simulink model "DC_SpeedControl"  (R2019b)
settings: Solver=VariableStepAuto  StartTime=0.0  StopTime=inf  RelTol=1e-3
libraries: powerlib x11, simulink x1
settings Model: Creator=Admin  LastModifiedBy=DELL
settings DataIOCC: ReturnWorkspaceOutputs=off
settings DebuggingCC: ArithmeticOperatorsInVariantConditions=warning
settings SFSimCC: SimUseLocalCustomCode=off  CustomCodeUndefinedFunction=UseInterfaceOnly
settings RTWCC: RTWUseLocalCustomCode=off

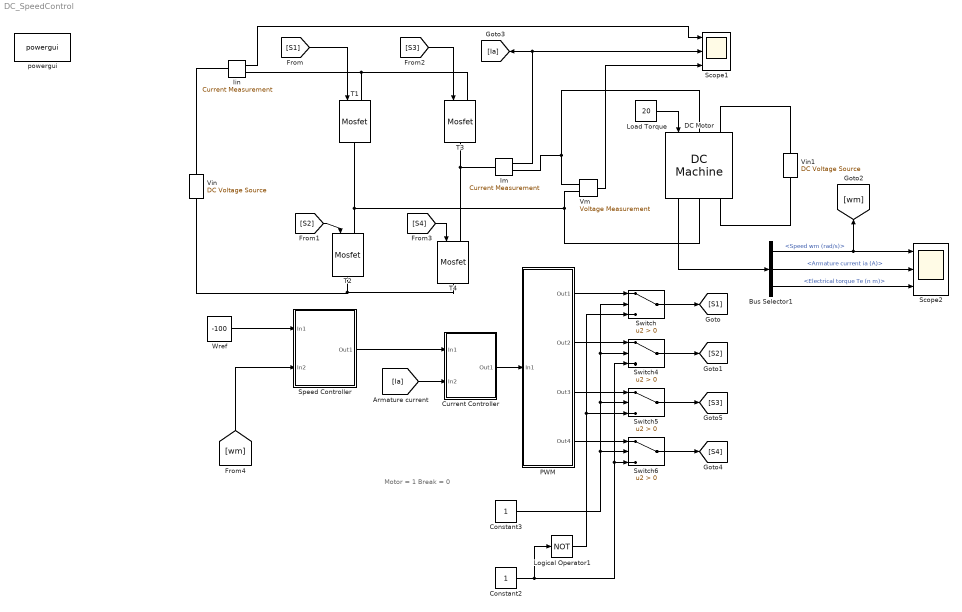
== system DC_SpeedControl ==
  note: Motor = 1
      | Break = 0
  Bus Selector1 : BusSelector  OutputSignals=Speed wm (rad/s),Armature current ia (A),Electrical torque Te (n m)
  Constant2 : Constant
  Constant3 : Constant
  Current Controller : Subsystem
  DC Motor : powerlib/Machines/DC Machine  PresetModel=02: 5HP 240V 1750RPM Field:150V  MechanicalLoad=Torque TL  FieldType=Wound  ShowDetailedParameters=on  MeasurementBus=off  RLa=[0.78 0.016]  RLf=[150 112.5]  Laf=1.234  MachineConstant=Torque constant (N.m/A)  Ke=1.8  Kt=1.8  J=0.05  Bm=0.01  Tf=0  w0=1  Ifinit=1  TsPowergui=0  TsBlock=-1
      settings: SourceProductName=Simscape Electrical
  Iin : powerlib/Measurements/Current Measurement  PhasorSimulation=off  OutputType=Complex  PSBequivalent=0
      settings: SourceProductName=Simscape Electrical
  Im : powerlib/Measurements/Current Measurement  PhasorSimulation=off  OutputType=Complex  PSBequivalent=0
      settings: SourceProductName=Simscape Electrical
  Load Torque : Constant  Value=20
  Logical Operator1 : Logic  Operator=NOT  AllPortsSameDT=off  OutDataTypeStr=boolean
  PWM : Subsystem
  Scope1 : Scope  NumInputPorts=3
  Scope2 : Scope  NumInputPorts=3
  Speed Controller : Subsystem
  Switch{,4..6} (4 alike) : Switch  Criteria=u2 > Threshold
  T{1..4} (4 alike) : powerlib/Power Electronics/Mosfet  Ron=0.1  Lon=0  Rd=0.01  Vfd=0  IC=0  Rs=1e5  Cs=inf  Measurements=off
      settings: SourceProductName=Simscape Electrical
  Vin : powerlib/Electrical Sources/DC Voltage Source  Amplitude=300  Measurements=None
      settings: SourceProductName=Simscape Electrical
  Vin1 : powerlib/Electrical Sources/DC Voltage Source  Amplitude=150  Measurements=None
      settings: SourceProductName=Simscape Electrical
  Vm : powerlib/Measurements/Voltage Measurement  PhasorSimulation=off  OutputType=Complex  PSBequivalent=0
      settings: SourceProductName=Simscape Electrical
  Wref : Constant  Value=-100  VectorParams1D=off  SampleTime=-1
  powergui : powerlib/powergui  Priority=1  SimulationMode=Continuous  SampleTime=50e-6  frequency=60  Iterations=50  frequencyindice=0  Pbase=100e6  ErrMax=1e-4  UnitsV=kV  UnitsW=MW  buscounter=0  FunctionMessages=off  echomessages=off  EnableUseOfTLC=off  CurrentSourceSwitches=off  DisableSnubberDevices=off  DisableRonSwitches=off  DisableVfSwitches=off  DisplayEquations=off  AutomaticDiscreteSolvers=off  SolverType=Tustin/Backward Euler (TBE)  Interpol=off  ExternalGateDelay=off  methode=off  Ts=100  x0status=blocks  SPID=on  SwTol=0  HookPort=off  NonlinearTolerance=1e-4  nMaxIteration=100  ContinueOnMaxIteration=off  RestoreLinks=warning  ResistiveCurrentMeasurement=off  Frange=[0:2:500]  Ylog=off  Xlog=on  ShowGrid=off  save=off  variable=ZData  structure=0  ZoomFFT=off  StartTime=0.0  cycles=1  DisplayStyle=1  fundamental=60  FreqAxis=off  MaxFrequency=1000  frequencyindicesteady=1  RmsSteady=1  display=off
      settings: SourceProductName=Simscape Electrical
  wires:
  Vm/1 -> Scope1/3
  Bus Selector1/1 -> [wm], Scope2/1  "<Speed wm (rad/s)>"
  Load Torque/1 -> DC Motor/1
  Bus Selector1/2 -> Scope2/2  "<Armature current ia (A)>"
  Iin/1 -> Scope1/1
  [S1] -> T1/1
  Bus Selector1/3 -> Scope2/3  "<Electrical torque Te (n m)>"
  [S3] -> T3/1
  DC Motor/1 -> Bus Selector1/1
  Im/1 -> [Ia], Scope1/2
  Wref/1 -> Speed Controller/1(In1)
  Speed Controller/1(Out1) -> Current Controller/1(In1)
  [Ia] -> Current Controller/2(In2)
  Current Controller/1(Out1) -> PWM/1(In1)
  [S4] -> T4/1
  [S2] -> T2/1
  PWM/1(Out1) -> Switch/1
  Switch/1 -> [S1]
  PWM/2(Out2) -> Switch4/1
  Switch4/1 -> [S2]
  PWM/3(Out3) -> Switch5/1
  Switch5/1 -> [S3]
  PWM/4(Out4) -> Switch6/1
  Switch6/1 -> [S4]
  Constant3/1 -> Switch5/2, Switch4/2, Switch/2, Switch6/2
  Constant2/1 -> Switch6/3, Switch4/3, Logical Operator1/1
  Logical Operator1/1 -> Switch5/3, Switch/3
  [wm] -> Speed Controller/2(In2)
  connections:
  T1/RConn1 -- Vm/LConn2 -- DC Motor/RConn1 -- T2/LConn1
  Im/RConn1 -- Vm/LConn1 -- DC Motor/LConn1
  Iin/RConn1 -- T1/LConn1 -- T3/LConn1
  Vin/LConn1 -- T4/RConn1 -- T2/RConn1
  Vin1/LConn1 -- DC Motor/RConn2
  Iin/LConn1 -- Vin/RConn1
  DC Motor/LConn2 -- Vin1/RConn1
  T4/LConn1 -- T3/RConn1 -- Im/LConn1

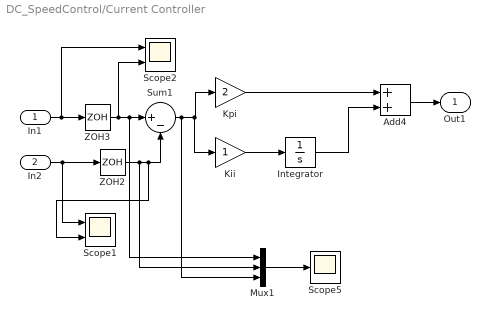
== system DC_SpeedControl/Current Controller ==
  In1 : Inport
  In2 : Inport  Port=2
  Add4 : Sum
  Integrator : Integrator
  Kii : Gain
  Kpi : Gain  Gain=2
  Mux1 : Mux  Inputs=3
  Scope1 : Scope  NumInputPorts=2
  Scope2 : Scope  NumInputPorts=2
  Scope5 : Scope
  Sum1 : Sum  Inputs=|+-
  ZOH2 : ZeroOrderHold  SampleTime=1e-4
  ZOH3 : ZeroOrderHold  SampleTime=1e-4
  Out1 : Outport  VectorParamsAs1DForOutWhenUnconnected=off
  wires:
  ZOH3/1 -> Scope2/2, Mux1/1, Sum1/1
  Kii/1 -> Integrator/1
  Sum1/1 -> Mux1/3, Kii/1, Kpi/1
  ZOH2/1 -> Mux1/2, Scope1/2, Sum1/2
  Mux1/1 -> Scope5/1
  Add4/1 -> Out1/1
  Kpi/1 -> Add4/1
  In1/1 -> Scope2/1, ZOH3/1
  In2/1 -> Scope1/1, ZOH2/1
  Integrator/1 -> Add4/2

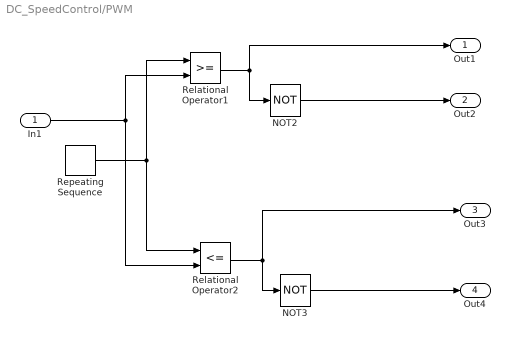
== system DC_SpeedControl/PWM ==
  In1 : Inport
  NOT2 : Logic  Operator=NOT  IconShape=distinctive  AllPortsSameDT=off  OutDataTypeStr=boolean
  NOT3 : Logic  Operator=NOT  IconShape=distinctive  AllPortsSameDT=off  OutDataTypeStr=boolean
  Relational Operator1 : RelationalOperator  OutDataTypeStr=boolean  RndMeth=Nearest
  Relational Operator2 : RelationalOperator  Operator=<=  OutDataTypeStr=boolean  RndMeth=Nearest
  Repeating Sequence : simulink/Sources/Repeating Sequence  rep_seq_t=[0 0.25 0.5 0.75 1]/1000  rep_seq_y=[0 1 0 -1 0]
  Out1 : Outport  VectorParamsAs1DForOutWhenUnconnected=off
  Out2 : Outport  Port=2  VectorParamsAs1DForOutWhenUnconnected=off
  Out3 : Outport  Port=3  VectorParamsAs1DForOutWhenUnconnected=off
  Out4 : Outport  Port=4  VectorParamsAs1DForOutWhenUnconnected=off
  wires:
  NOT3/1 -> Out4/1
  Repeating Sequence/1 -> Relational Operator1/1, Relational Operator2/1
  Relational Operator2/1 -> Out3/1, NOT3/1
  In1/1 -> Relational Operator1/2, Relational Operator2/2
  Relational Operator1/1 -> Out1/1, NOT2/1
  NOT2/1 -> Out2/1

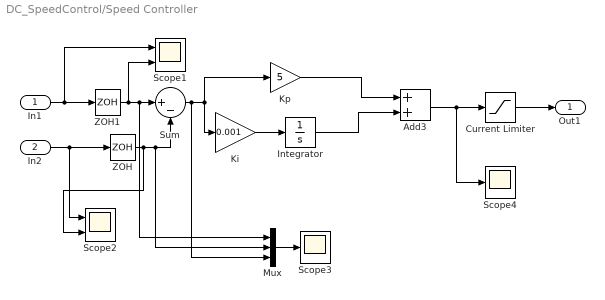
== system DC_SpeedControl/Speed Controller ==
  In1 : Inport
  In2 : Inport  Port=2
  Add3 : Sum
  Current Limiter : Saturate  UpperLimit=50  LowerLimit=0
  Integrator : Integrator
  Ki : Gain  Gain=0.001
  Kp : Gain  Gain=5
  Mux : Mux  Inputs=3
  Scope1 : Scope  NumInputPorts=2
  Scope2 : Scope  NumInputPorts=2
  Scope3 : Scope
  Scope4 : Scope
  Sum : Sum  Inputs=|+-
  ZOH : ZeroOrderHold  SampleTime=1e-4
  ZOH1 : ZeroOrderHold  SampleTime=1e-4
  Out1 : Outport  VectorParamsAs1DForOutWhenUnconnected=off
  wires:
  Sum/1 -> Mux/3, Ki/1, Kp/1
  Mux/1 -> Scope3/1
  Ki/1 -> Integrator/1
  ZOH/1 -> Scope2/2, Mux/2, Sum/2
  Add3/1 -> Scope4/1, Current Limiter/1
  ZOH1/1 -> Scope1/2, Mux/1, Sum/1
  Kp/1 -> Add3/1
  Current Limiter/1 -> Out1/1
  In1/1 -> Scope1/1, ZOH1/1
  In2/1 -> Scope2/1, ZOH/1
  Integrator/1 -> Add3/2
